simulink model "BAS_MPC_TV"  (R2018b)
settings: Solver=VariableStepAuto  StartTime=0.0  StopTime=10.0  RelTol=1e-3
values from neighbouring files (symbols this model uses):
  a = 1    [adaptive_mpc_tv.mat]
  b = 0.5    [adaptive_mpc_tv.mat]
  Izz = 100    [adaptive_mpc_tv.mat]
  M = 300    [adaptive_mpc_tv.mat]
  Rt = 0.226    [adaptive_mpc_tv.mat]
  track = 1.2    [adaptive_mpc_tv.mat]
  Ts = 0.02    [adaptive_mpc_tv.mat]
(part 2 of 2)

== system BAS_MPC_TV/For Iterator Subsystem1/function1/10layer_model/state_k_to_k+10 ==
  Fx : Inport
  Fy : Inport  Port=2
  statek : Inport  Port=3
  Add{,1,3..5,7} (6 alike) : Sum
  Add2 : Sum  Inputs=-+
  Add6 : Sum  Inputs=+--+-+
  Constant : Constant  Value=a
  Constant1 : Constant  Value=b
  Constant2 : Constant  Value=track
  Demux : Demux
  Demux1 : Demux
  Demux2 : Demux  Outputs=3
  Gain : Gain  Gain=0.5
  Multiply{,1..7} (8 alike) : Product
  Mux : Mux  Inputs=3
  Plus : Sum  Inputs=4
  Plus1 : Sum  Inputs=4
  Ts/Izz : Gain  Gain=Ts/Izz
  Ts/M : Gain  Gain=Ts/M
  Ts/M1 : Gain  Gain=Ts/M
  statek+1 : Outport
  wires:
  Demux2/2 -> Add3/1, Multiply/1
  Demux2/3 -> Multiply1/2, Multiply/2, Add7/1
  Multiply/1 -> Add/1
  Add/1 -> Ts/M/1
  Ts/M/1 -> Add1/2  "delta_Vx"
  Demux2/1 -> Add1/1, Multiply1/1
  Add1/1 -> Mux/1  "Vxk+1"
  Fx/1 -> Demux/1
  Demux/1 -> Multiply4/1, Plus/1  "Fx_FL"
  Demux/2 -> Multiply5/1, Plus/2  "Fx_FR"
  Demux/3 -> Multiply6/2, Plus/3  "Fx_RL"
  Demux/4 -> Plus/4, Multiply7/2  "Fx_RR"
  Plus/1 -> Add/2  "sumFx"
  Demux1/3 -> Add5/1, Plus1/3  "Fy_RL"
  Demux1/2 -> Add4/1, Plus1/2  "Fy_FR"
  Demux1/1 -> Add4/2, Plus1/1  "Fy_FL"
  Demux1/4 -> Add5/2, Plus1/4  "Fy_RR"
  Fy/1 -> Demux1/1
  Plus1/1 -> Add2/2  "sumFy"
  Multiply1/1 -> Add2/1
  Add2/1 -> Ts/M1/1
  Ts/M1/1 -> Add3/2  "delta_Vy"
  Add3/1 -> Mux/2  "Vyk+1"
  Add4/1 -> Multiply2/1
  Constant/1 -> Multiply2/2
  Multiply2/1 -> Add6/1
  Multiply3/1 -> Add6/2
  Constant1/1 -> Multiply3/2
  Add5/1 -> Multiply3/1
  Constant2/1 -> Gain/1
  Gain/1 -> Multiply7/1, Multiply4/2, Multiply5/2, Multiply6/1
  Multiply4/1 -> Add6/3
  Multiply5/1 -> Add6/4
  Multiply6/1 -> Add6/5
  Multiply7/1 -> Add6/6
  Add6/1 -> Ts/Izz/1
  Ts/Izz/1 -> Add7/2  "delta_yawrate"
  Add7/1 -> Mux/3  "yawratek+1"
  statek/1 -> Demux2/1
  Mux/1 -> statek+1/1

== system BAS_MPC_TV/For Iterator Subsystem1/function1/10layer_model/state_k_to_k+2 ==
  Fx : Inport
  Fy : Inport  Port=2
  statek : Inport  Port=3
  Add{,1,3..5,7} (6 alike) : Sum
  Add2 : Sum  Inputs=-+
  Add6 : Sum  Inputs=+--+-+
  Constant : Constant  Value=a
  Constant1 : Constant  Value=b
  Constant2 : Constant  Value=track
  Demux : Demux
  Demux1 : Demux
  Demux2 : Demux  Outputs=3
  Gain : Gain  Gain=0.5
  Multiply{,1..7} (8 alike) : Product
  Mux : Mux  Inputs=3
  Plus : Sum  Inputs=4
  Plus1 : Sum  Inputs=4
  Ts/Izz : Gain  Gain=Ts/Izz
  Ts/M : Gain  Gain=Ts/M
  Ts/M1 : Gain  Gain=Ts/M
  statek+1 : Outport
  wires:
  Demux2/2 -> Add3/1, Multiply/1
  Demux2/3 -> Multiply1/2, Multiply/2, Add7/1
  Multiply/1 -> Add/1
  Add/1 -> Ts/M/1
  Ts/M/1 -> Add1/2  "delta_Vx"
  Demux2/1 -> Add1/1, Multiply1/1
  Add1/1 -> Mux/1  "Vxk+1"
  Fx/1 -> Demux/1
  Demux/1 -> Multiply4/1, Plus/1  "Fx_FL"
  Demux/2 -> Multiply5/1, Plus/2  "Fx_FR"
  Demux/3 -> Multiply6/2, Plus/3  "Fx_RL"
  Demux/4 -> Plus/4, Multiply7/2  "Fx_RR"
  Plus/1 -> Add/2  "sumFx"
  Demux1/3 -> Add5/1, Plus1/3  "Fy_RL"
  Demux1/2 -> Add4/1, Plus1/2  "Fy_FR"
  Demux1/1 -> Add4/2, Plus1/1  "Fy_FL"
  Demux1/4 -> Add5/2, Plus1/4  "Fy_RR"
  Fy/1 -> Demux1/1
  Plus1/1 -> Add2/2  "sumFy"
  Multiply1/1 -> Add2/1
  Add2/1 -> Ts/M1/1
  Ts/M1/1 -> Add3/2  "delta_Vy"
  Add3/1 -> Mux/2  "Vyk+1"
  Add4/1 -> Multiply2/1
  Constant/1 -> Multiply2/2
  Multiply2/1 -> Add6/1
  Multiply3/1 -> Add6/2
  Constant1/1 -> Multiply3/2
  Add5/1 -> Multiply3/1
  Constant2/1 -> Gain/1
  Gain/1 -> Multiply7/1, Multiply4/2, Multiply5/2, Multiply6/1
  Multiply4/1 -> Add6/3
  Multiply5/1 -> Add6/4
  Multiply6/1 -> Add6/5
  Multiply7/1 -> Add6/6
  Add6/1 -> Ts/Izz/1
  Ts/Izz/1 -> Add7/2  "delta_yawrate"
  Add7/1 -> Mux/3  "yawratek+1"
  statek/1 -> Demux2/1
  Mux/1 -> statek+1/1

== system BAS_MPC_TV/For Iterator Subsystem1/function1/10layer_model/state_k_to_k+3 ==
  Fx : Inport
  Fy : Inport  Port=2
  statek : Inport  Port=3
  Add{,1,3..5,7} (6 alike) : Sum
  Add2 : Sum  Inputs=-+
  Add6 : Sum  Inputs=+--+-+
  Constant : Constant  Value=a
  Constant1 : Constant  Value=b
  Constant2 : Constant  Value=track
  Demux : Demux
  Demux1 : Demux
  Demux2 : Demux  Outputs=3
  Gain : Gain  Gain=0.5
  Multiply{,1..7} (8 alike) : Product
  Mux : Mux  Inputs=3
  Plus : Sum  Inputs=4
  Plus1 : Sum  Inputs=4
  Ts/Izz : Gain  Gain=Ts/Izz
  Ts/M : Gain  Gain=Ts/M
  Ts/M1 : Gain  Gain=Ts/M
  statek+1 : Outport
  wires:
  Demux2/2 -> Add3/1, Multiply/1
  Demux2/3 -> Multiply1/2, Multiply/2, Add7/1
  Multiply/1 -> Add/1
  Add/1 -> Ts/M/1
  Ts/M/1 -> Add1/2  "delta_Vx"
  Demux2/1 -> Add1/1, Multiply1/1
  Add1/1 -> Mux/1  "Vxk+1"
  Fx/1 -> Demux/1
  Demux/1 -> Multiply4/1, Plus/1  "Fx_FL"
  Demux/2 -> Multiply5/1, Plus/2  "Fx_FR"
  Demux/3 -> Multiply6/2, Plus/3  "Fx_RL"
  Demux/4 -> Plus/4, Multiply7/2  "Fx_RR"
  Plus/1 -> Add/2  "sumFx"
  Demux1/3 -> Add5/1, Plus1/3  "Fy_RL"
  Demux1/2 -> Add4/1, Plus1/2  "Fy_FR"
  Demux1/1 -> Add4/2, Plus1/1  "Fy_FL"
  Demux1/4 -> Add5/2, Plus1/4  "Fy_RR"
  Fy/1 -> Demux1/1
  Plus1/1 -> Add2/2  "sumFy"
  Multiply1/1 -> Add2/1
  Add2/1 -> Ts/M1/1
  Ts/M1/1 -> Add3/2  "delta_Vy"
  Add3/1 -> Mux/2  "Vyk+1"
  Add4/1 -> Multiply2/1
  Constant/1 -> Multiply2/2
  Multiply2/1 -> Add6/1
  Multiply3/1 -> Add6/2
  Constant1/1 -> Multiply3/2
  Add5/1 -> Multiply3/1
  Constant2/1 -> Gain/1
  Gain/1 -> Multiply7/1, Multiply4/2, Multiply5/2, Multiply6/1
  Multiply4/1 -> Add6/3
  Multiply5/1 -> Add6/4
  Multiply6/1 -> Add6/5
  Multiply7/1 -> Add6/6
  Add6/1 -> Ts/Izz/1
  Ts/Izz/1 -> Add7/2  "delta_yawrate"
  Add7/1 -> Mux/3  "yawratek+1"
  statek/1 -> Demux2/1
  Mux/1 -> statek+1/1

== system BAS_MPC_TV/For Iterator Subsystem1/function1/10layer_model/state_k_to_k+4 ==
  Fx : Inport
  Fy : Inport  Port=2
  statek : Inport  Port=3
  Add{,1,3..5,7} (6 alike) : Sum
  Add2 : Sum  Inputs=-+
  Add6 : Sum  Inputs=+--+-+
  Constant : Constant  Value=a
  Constant1 : Constant  Value=b
  Constant2 : Constant  Value=track
  Demux : Demux
  Demux1 : Demux
  Demux2 : Demux  Outputs=3
  Gain : Gain  Gain=0.5
  Multiply{,1..7} (8 alike) : Product
  Mux : Mux  Inputs=3
  Plus : Sum  Inputs=4
  Plus1 : Sum  Inputs=4
  Ts/Izz : Gain  Gain=Ts/Izz
  Ts/M : Gain  Gain=Ts/M
  Ts/M1 : Gain  Gain=Ts/M
  statek+1 : Outport
  wires:
  Demux2/2 -> Add3/1, Multiply/1
  Demux2/3 -> Multiply1/2, Multiply/2, Add7/1
  Multiply/1 -> Add/1
  Add/1 -> Ts/M/1
  Ts/M/1 -> Add1/2  "delta_Vx"
  Demux2/1 -> Add1/1, Multiply1/1
  Add1/1 -> Mux/1  "Vxk+1"
  Fx/1 -> Demux/1
  Demux/1 -> Multiply4/1, Plus/1  "Fx_FL"
  Demux/2 -> Multiply5/1, Plus/2  "Fx_FR"
  Demux/3 -> Multiply6/2, Plus/3  "Fx_RL"
  Demux/4 -> Plus/4, Multiply7/2  "Fx_RR"
  Plus/1 -> Add/2  "sumFx"
  Demux1/3 -> Add5/1, Plus1/3  "Fy_RL"
  Demux1/2 -> Add4/1, Plus1/2  "Fy_FR"
  Demux1/1 -> Add4/2, Plus1/1  "Fy_FL"
  Demux1/4 -> Add5/2, Plus1/4  "Fy_RR"
  Fy/1 -> Demux1/1
  Plus1/1 -> Add2/2  "sumFy"
  Multiply1/1 -> Add2/1
  Add2/1 -> Ts/M1/1
  Ts/M1/1 -> Add3/2  "delta_Vy"
  Add3/1 -> Mux/2  "Vyk+1"
  Add4/1 -> Multiply2/1
  Constant/1 -> Multiply2/2
  Multiply2/1 -> Add6/1
  Multiply3/1 -> Add6/2
  Constant1/1 -> Multiply3/2
  Add5/1 -> Multiply3/1
  Constant2/1 -> Gain/1
  Gain/1 -> Multiply7/1, Multiply4/2, Multiply5/2, Multiply6/1
  Multiply4/1 -> Add6/3
  Multiply5/1 -> Add6/4
  Multiply6/1 -> Add6/5
  Multiply7/1 -> Add6/6
  Add6/1 -> Ts/Izz/1
  Ts/Izz/1 -> Add7/2  "delta_yawrate"
  Add7/1 -> Mux/3  "yawratek+1"
  statek/1 -> Demux2/1
  Mux/1 -> statek+1/1

== system BAS_MPC_TV/For Iterator Subsystem1/function1/10layer_model/state_k_to_k+5 ==
  Fx : Inport
  Fy : Inport  Port=2
  statek : Inport  Port=3
  Add{,1,3..5,7} (6 alike) : Sum
  Add2 : Sum  Inputs=-+
  Add6 : Sum  Inputs=+--+-+
  Constant : Constant  Value=a
  Constant1 : Constant  Value=b
  Constant2 : Constant  Value=track
  Demux : Demux
  Demux1 : Demux
  Demux2 : Demux  Outputs=3
  Gain : Gain  Gain=0.5
  Multiply{,1..7} (8 alike) : Product
  Mux : Mux  Inputs=3
  Plus : Sum  Inputs=4
  Plus1 : Sum  Inputs=4
  Ts/Izz : Gain  Gain=Ts/Izz
  Ts/M : Gain  Gain=Ts/M
  Ts/M1 : Gain  Gain=Ts/M
  statek+1 : Outport
  wires:
  Demux2/2 -> Add3/1, Multiply/1
  Demux2/3 -> Multiply1/2, Multiply/2, Add7/1
  Multiply/1 -> Add/1
  Add/1 -> Ts/M/1
  Ts/M/1 -> Add1/2  "delta_Vx"
  Demux2/1 -> Add1/1, Multiply1/1
  Add1/1 -> Mux/1  "Vxk+1"
  Fx/1 -> Demux/1
  Demux/1 -> Multiply4/1, Plus/1  "Fx_FL"
  Demux/2 -> Multiply5/1, Plus/2  "Fx_FR"
  Demux/3 -> Multiply6/2, Plus/3  "Fx_RL"
  Demux/4 -> Plus/4, Multiply7/2  "Fx_RR"
  Plus/1 -> Add/2  "sumFx"
  Demux1/3 -> Add5/1, Plus1/3  "Fy_RL"
  Demux1/2 -> Add4/1, Plus1/2  "Fy_FR"
  Demux1/1 -> Add4/2, Plus1/1  "Fy_FL"
  Demux1/4 -> Add5/2, Plus1/4  "Fy_RR"
  Fy/1 -> Demux1/1
  Plus1/1 -> Add2/2  "sumFy"
  Multiply1/1 -> Add2/1
  Add2/1 -> Ts/M1/1
  Ts/M1/1 -> Add3/2  "delta_Vy"
  Add3/1 -> Mux/2  "Vyk+1"
  Add4/1 -> Multiply2/1
  Constant/1 -> Multiply2/2
  Multiply2/1 -> Add6/1
  Multiply3/1 -> Add6/2
  Constant1/1 -> Multiply3/2
  Add5/1 -> Multiply3/1
  Constant2/1 -> Gain/1
  Gain/1 -> Multiply7/1, Multiply4/2, Multiply5/2, Multiply6/1
  Multiply4/1 -> Add6/3
  Multiply5/1 -> Add6/4
  Multiply6/1 -> Add6/5
  Multiply7/1 -> Add6/6
  Add6/1 -> Ts/Izz/1
  Ts/Izz/1 -> Add7/2  "delta_yawrate"
  Add7/1 -> Mux/3  "yawratek+1"
  statek/1 -> Demux2/1
  Mux/1 -> statek+1/1

== system BAS_MPC_TV/For Iterator Subsystem1/function1/10layer_model/state_k_to_k+6 ==
  Fx : Inport
  Fy : Inport  Port=2
  statek : Inport  Port=3
  Add{,1,3..5,7} (6 alike) : Sum
  Add2 : Sum  Inputs=-+
  Add6 : Sum  Inputs=+--+-+
  Constant : Constant  Value=a
  Constant1 : Constant  Value=b
  Constant2 : Constant  Value=track
  Demux : Demux
  Demux1 : Demux
  Demux2 : Demux  Outputs=3
  Gain : Gain  Gain=0.5
  Multiply{,1..7} (8 alike) : Product
  Mux : Mux  Inputs=3
  Plus : Sum  Inputs=4
  Plus1 : Sum  Inputs=4
  Ts/Izz : Gain  Gain=Ts/Izz
  Ts/M : Gain  Gain=Ts/M
  Ts/M1 : Gain  Gain=Ts/M
  statek+1 : Outport
  wires:
  Demux2/2 -> Add3/1, Multiply/1
  Demux2/3 -> Multiply1/2, Multiply/2, Add7/1
  Multiply/1 -> Add/1
  Add/1 -> Ts/M/1
  Ts/M/1 -> Add1/2  "delta_Vx"
  Demux2/1 -> Add1/1, Multiply1/1
  Add1/1 -> Mux/1  "Vxk+1"
  Fx/1 -> Demux/1
  Demux/1 -> Multiply4/1, Plus/1  "Fx_FL"
  Demux/2 -> Multiply5/1, Plus/2  "Fx_FR"
  Demux/3 -> Multiply6/2, Plus/3  "Fx_RL"
  Demux/4 -> Plus/4, Multiply7/2  "Fx_RR"
  Plus/1 -> Add/2  "sumFx"
  Demux1/3 -> Add5/1, Plus1/3  "Fy_RL"
  Demux1/2 -> Add4/1, Plus1/2  "Fy_FR"
  Demux1/1 -> Add4/2, Plus1/1  "Fy_FL"
  Demux1/4 -> Add5/2, Plus1/4  "Fy_RR"
  Fy/1 -> Demux1/1
  Plus1/1 -> Add2/2  "sumFy"
  Multiply1/1 -> Add2/1
  Add2/1 -> Ts/M1/1
  Ts/M1/1 -> Add3/2  "delta_Vy"
  Add3/1 -> Mux/2  "Vyk+1"
  Add4/1 -> Multiply2/1
  Constant/1 -> Multiply2/2
  Multiply2/1 -> Add6/1
  Multiply3/1 -> Add6/2
  Constant1/1 -> Multiply3/2
  Add5/1 -> Multiply3/1
  Constant2/1 -> Gain/1
  Gain/1 -> Multiply7/1, Multiply4/2, Multiply5/2, Multiply6/1
  Multiply4/1 -> Add6/3
  Multiply5/1 -> Add6/4
  Multiply6/1 -> Add6/5
  Multiply7/1 -> Add6/6
  Add6/1 -> Ts/Izz/1
  Ts/Izz/1 -> Add7/2  "delta_yawrate"
  Add7/1 -> Mux/3  "yawratek+1"
  statek/1 -> Demux2/1
  Mux/1 -> statek+1/1

== system BAS_MPC_TV/For Iterator Subsystem1/function1/10layer_model/state_k_to_k+7 ==
  Fx : Inport
  Fy : Inport  Port=2
  statek : Inport  Port=3
  Add{,1,3..5,7} (6 alike) : Sum
  Add2 : Sum  Inputs=-+
  Add6 : Sum  Inputs=+--+-+
  Constant : Constant  Value=a
  Constant1 : Constant  Value=b
  Constant2 : Constant  Value=track
  Demux : Demux
  Demux1 : Demux
  Demux2 : Demux  Outputs=3
  Gain : Gain  Gain=0.5
  Multiply{,1..7} (8 alike) : Product
  Mux : Mux  Inputs=3
  Plus : Sum  Inputs=4
  Plus1 : Sum  Inputs=4
  Ts/Izz : Gain  Gain=Ts/Izz
  Ts/M : Gain  Gain=Ts/M
  Ts/M1 : Gain  Gain=Ts/M
  statek+1 : Outport
  wires:
  Demux2/2 -> Add3/1, Multiply/1
  Demux2/3 -> Multiply1/2, Multiply/2, Add7/1
  Multiply/1 -> Add/1
  Add/1 -> Ts/M/1
  Ts/M/1 -> Add1/2  "delta_Vx"
  Demux2/1 -> Add1/1, Multiply1/1
  Add1/1 -> Mux/1  "Vxk+1"
  Fx/1 -> Demux/1
  Demux/1 -> Multiply4/1, Plus/1  "Fx_FL"
  Demux/2 -> Multiply5/1, Plus/2  "Fx_FR"
  Demux/3 -> Multiply6/2, Plus/3  "Fx_RL"
  Demux/4 -> Plus/4, Multiply7/2  "Fx_RR"
  Plus/1 -> Add/2  "sumFx"
  Demux1/3 -> Add5/1, Plus1/3  "Fy_RL"
  Demux1/2 -> Add4/1, Plus1/2  "Fy_FR"
  Demux1/1 -> Add4/2, Plus1/1  "Fy_FL"
  Demux1/4 -> Add5/2, Plus1/4  "Fy_RR"
  Fy/1 -> Demux1/1
  Plus1/1 -> Add2/2  "sumFy"
  Multiply1/1 -> Add2/1
  Add2/1 -> Ts/M1/1
  Ts/M1/1 -> Add3/2  "delta_Vy"
  Add3/1 -> Mux/2  "Vyk+1"
  Add4/1 -> Multiply2/1
  Constant/1 -> Multiply2/2
  Multiply2/1 -> Add6/1
  Multiply3/1 -> Add6/2
  Constant1/1 -> Multiply3/2
  Add5/1 -> Multiply3/1
  Constant2/1 -> Gain/1
  Gain/1 -> Multiply7/1, Multiply4/2, Multiply5/2, Multiply6/1
  Multiply4/1 -> Add6/3
  Multiply5/1 -> Add6/4
  Multiply6/1 -> Add6/5
  Multiply7/1 -> Add6/6
  Add6/1 -> Ts/Izz/1
  Ts/Izz/1 -> Add7/2  "delta_yawrate"
  Add7/1 -> Mux/3  "yawratek+1"
  statek/1 -> Demux2/1
  Mux/1 -> statek+1/1

== system BAS_MPC_TV/For Iterator Subsystem1/function1/10layer_model/state_k_to_k+8 ==
  Fx : Inport
  Fy : Inport  Port=2
  statek : Inport  Port=3
  Add{,1,3..5,7} (6 alike) : Sum
  Add2 : Sum  Inputs=-+
  Add6 : Sum  Inputs=+--+-+
  Constant : Constant  Value=a
  Constant1 : Constant  Value=b
  Constant2 : Constant  Value=track
  Demux : Demux
  Demux1 : Demux
  Demux2 : Demux  Outputs=3
  Gain : Gain  Gain=0.5
  Multiply{,1..7} (8 alike) : Product
  Mux : Mux  Inputs=3
  Plus : Sum  Inputs=4
  Plus1 : Sum  Inputs=4
  Ts/Izz : Gain  Gain=Ts/Izz
  Ts/M : Gain  Gain=Ts/M
  Ts/M1 : Gain  Gain=Ts/M
  statek+1 : Outport
  wires:
  Demux2/2 -> Add3/1, Multiply/1
  Demux2/3 -> Multiply1/2, Multiply/2, Add7/1
  Multiply/1 -> Add/1
  Add/1 -> Ts/M/1
  Ts/M/1 -> Add1/2  "delta_Vx"
  Demux2/1 -> Add1/1, Multiply1/1
  Add1/1 -> Mux/1  "Vxk+1"
  Fx/1 -> Demux/1
  Demux/1 -> Multiply4/1, Plus/1  "Fx_FL"
  Demux/2 -> Multiply5/1, Plus/2  "Fx_FR"
  Demux/3 -> Multiply6/2, Plus/3  "Fx_RL"
  Demux/4 -> Plus/4, Multiply7/2  "Fx_RR"
  Plus/1 -> Add/2  "sumFx"
  Demux1/3 -> Add5/1, Plus1/3  "Fy_RL"
  Demux1/2 -> Add4/1, Plus1/2  "Fy_FR"
  Demux1/1 -> Add4/2, Plus1/1  "Fy_FL"
  Demux1/4 -> Add5/2, Plus1/4  "Fy_RR"
  Fy/1 -> Demux1/1
  Plus1/1 -> Add2/2  "sumFy"
  Multiply1/1 -> Add2/1
  Add2/1 -> Ts/M1/1
  Ts/M1/1 -> Add3/2  "delta_Vy"
  Add3/1 -> Mux/2  "Vyk+1"
  Add4/1 -> Multiply2/1
  Constant/1 -> Multiply2/2
  Multiply2/1 -> Add6/1
  Multiply3/1 -> Add6/2
  Constant1/1 -> Multiply3/2
  Add5/1 -> Multiply3/1
  Constant2/1 -> Gain/1
  Gain/1 -> Multiply7/1, Multiply4/2, Multiply5/2, Multiply6/1
  Multiply4/1 -> Add6/3
  Multiply5/1 -> Add6/4
  Multiply6/1 -> Add6/5
  Multiply7/1 -> Add6/6
  Add6/1 -> Ts/Izz/1
  Ts/Izz/1 -> Add7/2  "delta_yawrate"
  Add7/1 -> Mux/3  "yawratek+1"
  statek/1 -> Demux2/1
  Mux/1 -> statek+1/1

== system BAS_MPC_TV/For Iterator Subsystem1/function1/10layer_model/state_k_to_k+9 ==
  Fx : Inport
  Fy : Inport  Port=2
  statek : Inport  Port=3
  Add{,1,3..5,7} (6 alike) : Sum
  Add2 : Sum  Inputs=-+
  Add6 : Sum  Inputs=+--+-+
  Constant : Constant  Value=a
  Constant1 : Constant  Value=b
  Constant2 : Constant  Value=track
  Demux : Demux
  Demux1 : Demux
  Demux2 : Demux  Outputs=3
  Gain : Gain  Gain=0.5
  Multiply{,1..7} (8 alike) : Product
  Mux : Mux  Inputs=3
  Plus : Sum  Inputs=4
  Plus1 : Sum  Inputs=4
  Ts/Izz : Gain  Gain=Ts/Izz
  Ts/M : Gain  Gain=Ts/M
  Ts/M1 : Gain  Gain=Ts/M
  statek+1 : Outport
  wires:
  Demux2/2 -> Add3/1, Multiply/1
  Demux2/3 -> Multiply1/2, Multiply/2, Add7/1
  Multiply/1 -> Add/1
  Add/1 -> Ts/M/1
  Ts/M/1 -> Add1/2  "delta_Vx"
  Demux2/1 -> Add1/1, Multiply1/1
  Add1/1 -> Mux/1  "Vxk+1"
  Fx/1 -> Demux/1
  Demux/1 -> Multiply4/1, Plus/1  "Fx_FL"
  Demux/2 -> Multiply5/1, Plus/2  "Fx_FR"
  Demux/3 -> Multiply6/2, Plus/3  "Fx_RL"
  Demux/4 -> Plus/4, Multiply7/2  "Fx_RR"
  Plus/1 -> Add/2  "sumFx"
  Demux1/3 -> Add5/1, Plus1/3  "Fy_RL"
  Demux1/2 -> Add4/1, Plus1/2  "Fy_FR"
  Demux1/1 -> Add4/2, Plus1/1  "Fy_FL"
  Demux1/4 -> Add5/2, Plus1/4  "Fy_RR"
  Fy/1 -> Demux1/1
  Plus1/1 -> Add2/2  "sumFy"
  Multiply1/1 -> Add2/1
  Add2/1 -> Ts/M1/1
  Ts/M1/1 -> Add3/2  "delta_Vy"
  Add3/1 -> Mux/2  "Vyk+1"
  Add4/1 -> Multiply2/1
  Constant/1 -> Multiply2/2
  Multiply2/1 -> Add6/1
  Multiply3/1 -> Add6/2
  Constant1/1 -> Multiply3/2
  Add5/1 -> Multiply3/1
  Constant2/1 -> Gain/1
  Gain/1 -> Multiply7/1, Multiply4/2, Multiply5/2, Multiply6/1
  Multiply4/1 -> Add6/3
  Multiply5/1 -> Add6/4
  Multiply6/1 -> Add6/5
  Multiply7/1 -> Add6/6
  Add6/1 -> Ts/Izz/1
  Ts/Izz/1 -> Add7/2  "delta_yawrate"
  Add7/1 -> Mux/3  "yawratek+1"
  statek/1 -> Demux2/1
  Mux/1 -> statek+1/1

== system BAS_MPC_TV/For Iterator Subsystem1/function2/10layer_model/state_k_to_k+1 ==
  Fx : Inport
  Fy : Inport  Port=2
  statek : Inport  Port=3
  Add{,1,3..5,7} (6 alike) : Sum
  Add2 : Sum  Inputs=-+
  Add6 : Sum  Inputs=+--+-+
  Constant : Constant  Value=a
  Constant1 : Constant  Value=b
  Constant2 : Constant  Value=track
  Demux : Demux
  Demux1 : Demux
  Demux2 : Demux  Outputs=3
  Gain : Gain  Gain=0.5
  Multiply{,1..7} (8 alike) : Product
  Mux : Mux  Inputs=3
  Plus : Sum  Inputs=4
  Plus1 : Sum  Inputs=4
  Ts/Izz : Gain  Gain=Ts/Izz
  Ts/M : Gain  Gain=Ts/M
  Ts/M1 : Gain  Gain=Ts/M
  statek+1 : Outport
  wires:
  Demux2/2 -> Add3/1, Multiply/1
  Demux2/3 -> Multiply1/2, Multiply/2, Add7/1
  Multiply/1 -> Add/1
  Add/1 -> Ts/M/1
  Ts/M/1 -> Add1/2  "delta_Vx"
  Demux2/1 -> Add1/1, Multiply1/1
  Add1/1 -> Mux/1  "Vxk+1"
  Fx/1 -> Demux/1
  Demux/1 -> Multiply4/1, Plus/1  "Fx_FL"
  Demux/2 -> Multiply5/1, Plus/2  "Fx_FR"
  Demux/3 -> Multiply6/2, Plus/3  "Fx_RL"
  Demux/4 -> Plus/4, Multiply7/2  "Fx_RR"
  Plus/1 -> Add/2  "sumFx"
  Demux1/3 -> Add5/1, Plus1/3  "Fy_RL"
  Demux1/2 -> Add4/1, Plus1/2  "Fy_FR"
  Demux1/1 -> Add4/2, Plus1/1  "Fy_FL"
  Demux1/4 -> Add5/2, Plus1/4  "Fy_RR"
  Fy/1 -> Demux1/1
  Plus1/1 -> Add2/2  "sumFy"
  Multiply1/1 -> Add2/1
  Add2/1 -> Ts/M1/1
  Ts/M1/1 -> Add3/2  "delta_Vy"
  Add3/1 -> Mux/2  "Vyk+1"
  Add4/1 -> Multiply2/1
  Constant/1 -> Multiply2/2
  Multiply2/1 -> Add6/1
  Multiply3/1 -> Add6/2
  Constant1/1 -> Multiply3/2
  Add5/1 -> Multiply3/1
  Constant2/1 -> Gain/1
  Gain/1 -> Multiply7/1, Multiply4/2, Multiply5/2, Multiply6/1
  Multiply4/1 -> Add6/3
  Multiply5/1 -> Add6/4
  Multiply6/1 -> Add6/5
  Multiply7/1 -> Add6/6
  Add6/1 -> Ts/Izz/1
  Ts/Izz/1 -> Add7/2  "delta_yawrate"
  Add7/1 -> Mux/3  "yawratek+1"
  statek/1 -> Demux2/1
  Mux/1 -> statek+1/1

== system BAS_MPC_TV/For Iterator Subsystem1/function2/10layer_model/state_k_to_k+10 ==
  Fx : Inport
  Fy : Inport  Port=2
  statek : Inport  Port=3
  Add{,1,3..5,7} (6 alike) : Sum
  Add2 : Sum  Inputs=-+
  Add6 : Sum  Inputs=+--+-+
  Constant : Constant  Value=a
  Constant1 : Constant  Value=b
  Constant2 : Constant  Value=track
  Demux : Demux
  Demux1 : Demux
  Demux2 : Demux  Outputs=3
  Gain : Gain  Gain=0.5
  Multiply{,1..7} (8 alike) : Product
  Mux : Mux  Inputs=3
  Plus : Sum  Inputs=4
  Plus1 : Sum  Inputs=4
  Ts/Izz : Gain  Gain=Ts/Izz
  Ts/M : Gain  Gain=Ts/M
  Ts/M1 : Gain  Gain=Ts/M
  statek+1 : Outport
  wires:
  Demux2/2 -> Add3/1, Multiply/1
  Demux2/3 -> Multiply1/2, Multiply/2, Add7/1
  Multiply/1 -> Add/1
  Add/1 -> Ts/M/1
  Ts/M/1 -> Add1/2  "delta_Vx"
  Demux2/1 -> Add1/1, Multiply1/1
  Add1/1 -> Mux/1  "Vxk+1"
  Fx/1 -> Demux/1
  Demux/1 -> Multiply4/1, Plus/1  "Fx_FL"
  Demux/2 -> Multiply5/1, Plus/2  "Fx_FR"
  Demux/3 -> Multiply6/2, Plus/3  "Fx_RL"
  Demux/4 -> Plus/4, Multiply7/2  "Fx_RR"
  Plus/1 -> Add/2  "sumFx"
  Demux1/3 -> Add5/1, Plus1/3  "Fy_RL"
  Demux1/2 -> Add4/1, Plus1/2  "Fy_FR"
  Demux1/1 -> Add4/2, Plus1/1  "Fy_FL"
  Demux1/4 -> Add5/2, Plus1/4  "Fy_RR"
  Fy/1 -> Demux1/1
  Plus1/1 -> Add2/2  "sumFy"
  Multiply1/1 -> Add2/1
  Add2/1 -> Ts/M1/1
  Ts/M1/1 -> Add3/2  "delta_Vy"
  Add3/1 -> Mux/2  "Vyk+1"
  Add4/1 -> Multiply2/1
  Constant/1 -> Multiply2/2
  Multiply2/1 -> Add6/1
  Multiply3/1 -> Add6/2
  Constant1/1 -> Multiply3/2
  Add5/1 -> Multiply3/1
  Constant2/1 -> Gain/1
  Gain/1 -> Multiply7/1, Multiply4/2, Multiply5/2, Multiply6/1
  Multiply4/1 -> Add6/3
  Multiply5/1 -> Add6/4
  Multiply6/1 -> Add6/5
  Multiply7/1 -> Add6/6
  Add6/1 -> Ts/Izz/1
  Ts/Izz/1 -> Add7/2  "delta_yawrate"
  Add7/1 -> Mux/3  "yawratek+1"
  statek/1 -> Demux2/1
  Mux/1 -> statek+1/1

== system BAS_MPC_TV/For Iterator Subsystem1/function2/10layer_model/state_k_to_k+2 ==
  Fx : Inport
  Fy : Inport  Port=2
  statek : Inport  Port=3
  Add{,1,3..5,7} (6 alike) : Sum
  Add2 : Sum  Inputs=-+
  Add6 : Sum  Inputs=+--+-+
  Constant : Constant  Value=a
  Constant1 : Constant  Value=b
  Constant2 : Constant  Value=track
  Demux : Demux
  Demux1 : Demux
  Demux2 : Demux  Outputs=3
  Gain : Gain  Gain=0.5
  Multiply{,1..7} (8 alike) : Product
  Mux : Mux  Inputs=3
  Plus : Sum  Inputs=4
  Plus1 : Sum  Inputs=4
  Ts/Izz : Gain  Gain=Ts/Izz
  Ts/M : Gain  Gain=Ts/M
  Ts/M1 : Gain  Gain=Ts/M
  statek+1 : Outport
  wires:
  Demux2/2 -> Add3/1, Multiply/1
  Demux2/3 -> Multiply1/2, Multiply/2, Add7/1
  Multiply/1 -> Add/1
  Add/1 -> Ts/M/1
  Ts/M/1 -> Add1/2  "delta_Vx"
  Demux2/1 -> Add1/1, Multiply1/1
  Add1/1 -> Mux/1  "Vxk+1"
  Fx/1 -> Demux/1
  Demux/1 -> Multiply4/1, Plus/1  "Fx_FL"
  Demux/2 -> Multiply5/1, Plus/2  "Fx_FR"
  Demux/3 -> Multiply6/2, Plus/3  "Fx_RL"
  Demux/4 -> Plus/4, Multiply7/2  "Fx_RR"
  Plus/1 -> Add/2  "sumFx"
  Demux1/3 -> Add5/1, Plus1/3  "Fy_RL"
  Demux1/2 -> Add4/1, Plus1/2  "Fy_FR"
  Demux1/1 -> Add4/2, Plus1/1  "Fy_FL"
  Demux1/4 -> Add5/2, Plus1/4  "Fy_RR"
  Fy/1 -> Demux1/1
  Plus1/1 -> Add2/2  "sumFy"
  Multiply1/1 -> Add2/1
  Add2/1 -> Ts/M1/1
  Ts/M1/1 -> Add3/2  "delta_Vy"
  Add3/1 -> Mux/2  "Vyk+1"
  Add4/1 -> Multiply2/1
  Constant/1 -> Multiply2/2
  Multiply2/1 -> Add6/1
  Multiply3/1 -> Add6/2
  Constant1/1 -> Multiply3/2
  Add5/1 -> Multiply3/1
  Constant2/1 -> Gain/1
  Gain/1 -> Multiply7/1, Multiply4/2, Multiply5/2, Multiply6/1
  Multiply4/1 -> Add6/3
  Multiply5/1 -> Add6/4
  Multiply6/1 -> Add6/5
  Multiply7/1 -> Add6/6
  Add6/1 -> Ts/Izz/1
  Ts/Izz/1 -> Add7/2  "delta_yawrate"
  Add7/1 -> Mux/3  "yawratek+1"
  statek/1 -> Demux2/1
  Mux/1 -> statek+1/1

== system BAS_MPC_TV/For Iterator Subsystem1/function2/10layer_model/state_k_to_k+3 ==
  Fx : Inport
  Fy : Inport  Port=2
  statek : Inport  Port=3
  Add{,1,3..5,7} (6 alike) : Sum
  Add2 : Sum  Inputs=-+
  Add6 : Sum  Inputs=+--+-+
  Constant : Constant  Value=a
  Constant1 : Constant  Value=b
  Constant2 : Constant  Value=track
  Demux : Demux
  Demux1 : Demux
  Demux2 : Demux  Outputs=3
  Gain : Gain  Gain=0.5
  Multiply{,1..7} (8 alike) : Product
  Mux : Mux  Inputs=3
  Plus : Sum  Inputs=4
  Plus1 : Sum  Inputs=4
  Ts/Izz : Gain  Gain=Ts/Izz
  Ts/M : Gain  Gain=Ts/M
  Ts/M1 : Gain  Gain=Ts/M
  statek+1 : Outport
  wires:
  Demux2/2 -> Add3/1, Multiply/1
  Demux2/3 -> Multiply1/2, Multiply/2, Add7/1
  Multiply/1 -> Add/1
  Add/1 -> Ts/M/1
  Ts/M/1 -> Add1/2  "delta_Vx"
  Demux2/1 -> Add1/1, Multiply1/1
  Add1/1 -> Mux/1  "Vxk+1"
  Fx/1 -> Demux/1
  Demux/1 -> Multiply4/1, Plus/1  "Fx_FL"
  Demux/2 -> Multiply5/1, Plus/2  "Fx_FR"
  Demux/3 -> Multiply6/2, Plus/3  "Fx_RL"
  Demux/4 -> Plus/4, Multiply7/2  "Fx_RR"
  Plus/1 -> Add/2  "sumFx"
  Demux1/3 -> Add5/1, Plus1/3  "Fy_RL"
  Demux1/2 -> Add4/1, Plus1/2  "Fy_FR"
  Demux1/1 -> Add4/2, Plus1/1  "Fy_FL"
  Demux1/4 -> Add5/2, Plus1/4  "Fy_RR"
  Fy/1 -> Demux1/1
  Plus1/1 -> Add2/2  "sumFy"
  Multiply1/1 -> Add2/1
  Add2/1 -> Ts/M1/1
  Ts/M1/1 -> Add3/2  "delta_Vy"
  Add3/1 -> Mux/2  "Vyk+1"
  Add4/1 -> Multiply2/1
  Constant/1 -> Multiply2/2
  Multiply2/1 -> Add6/1
  Multiply3/1 -> Add6/2
  Constant1/1 -> Multiply3/2
  Add5/1 -> Multiply3/1
  Constant2/1 -> Gain/1
  Gain/1 -> Multiply7/1, Multiply4/2, Multiply5/2, Multiply6/1
  Multiply4/1 -> Add6/3
  Multiply5/1 -> Add6/4
  Multiply6/1 -> Add6/5
  Multiply7/1 -> Add6/6
  Add6/1 -> Ts/Izz/1
  Ts/Izz/1 -> Add7/2  "delta_yawrate"
  Add7/1 -> Mux/3  "yawratek+1"
  statek/1 -> Demux2/1
  Mux/1 -> statek+1/1

== system BAS_MPC_TV/For Iterator Subsystem1/function2/10layer_model/state_k_to_k+4 ==
  Fx : Inport
  Fy : Inport  Port=2
  statek : Inport  Port=3
  Add{,1,3..5,7} (6 alike) : Sum
  Add2 : Sum  Inputs=-+
  Add6 : Sum  Inputs=+--+-+
  Constant : Constant  Value=a
  Constant1 : Constant  Value=b
  Constant2 : Constant  Value=track
  Demux : Demux
  Demux1 : Demux
  Demux2 : Demux  Outputs=3
  Gain : Gain  Gain=0.5
  Multiply{,1..7} (8 alike) : Product
  Mux : Mux  Inputs=3
  Plus : Sum  Inputs=4
  Plus1 : Sum  Inputs=4
  Ts/Izz : Gain  Gain=Ts/Izz
  Ts/M : Gain  Gain=Ts/M
  Ts/M1 : Gain  Gain=Ts/M
  statek+1 : Outport
  wires:
  Demux2/2 -> Add3/1, Multiply/1
  Demux2/3 -> Multiply1/2, Multiply/2, Add7/1
  Multiply/1 -> Add/1
  Add/1 -> Ts/M/1
  Ts/M/1 -> Add1/2  "delta_Vx"
  Demux2/1 -> Add1/1, Multiply1/1
  Add1/1 -> Mux/1  "Vxk+1"
  Fx/1 -> Demux/1
  Demux/1 -> Multiply4/1, Plus/1  "Fx_FL"
  Demux/2 -> Multiply5/1, Plus/2  "Fx_FR"
  Demux/3 -> Multiply6/2, Plus/3  "Fx_RL"
  Demux/4 -> Plus/4, Multiply7/2  "Fx_RR"
  Plus/1 -> Add/2  "sumFx"
  Demux1/3 -> Add5/1, Plus1/3  "Fy_RL"
  Demux1/2 -> Add4/1, Plus1/2  "Fy_FR"
  Demux1/1 -> Add4/2, Plus1/1  "Fy_FL"
  Demux1/4 -> Add5/2, Plus1/4  "Fy_RR"
  Fy/1 -> Demux1/1
  Plus1/1 -> Add2/2  "sumFy"
  Multiply1/1 -> Add2/1
  Add2/1 -> Ts/M1/1
  Ts/M1/1 -> Add3/2  "delta_Vy"
  Add3/1 -> Mux/2  "Vyk+1"
  Add4/1 -> Multiply2/1
  Constant/1 -> Multiply2/2
  Multiply2/1 -> Add6/1
  Multiply3/1 -> Add6/2
  Constant1/1 -> Multiply3/2
  Add5/1 -> Multiply3/1
  Constant2/1 -> Gain/1
  Gain/1 -> Multiply7/1, Multiply4/2, Multiply5/2, Multiply6/1
  Multiply4/1 -> Add6/3
  Multiply5/1 -> Add6/4
  Multiply6/1 -> Add6/5
  Multiply7/1 -> Add6/6
  Add6/1 -> Ts/Izz/1
  Ts/Izz/1 -> Add7/2  "delta_yawrate"
  Add7/1 -> Mux/3  "yawratek+1"
  statek/1 -> Demux2/1
  Mux/1 -> statek+1/1

== system BAS_MPC_TV/For Iterator Subsystem1/function2/10layer_model/state_k_to_k+5 ==
  Fx : Inport
  Fy : Inport  Port=2
  statek : Inport  Port=3
  Add{,1,3..5,7} (6 alike) : Sum
  Add2 : Sum  Inputs=-+
  Add6 : Sum  Inputs=+--+-+
  Constant : Constant  Value=a
  Constant1 : Constant  Value=b
  Constant2 : Constant  Value=track
  Demux : Demux
  Demux1 : Demux
  Demux2 : Demux  Outputs=3
  Gain : Gain  Gain=0.5
  Multiply{,1..7} (8 alike) : Product
  Mux : Mux  Inputs=3
  Plus : Sum  Inputs=4
  Plus1 : Sum  Inputs=4
  Ts/Izz : Gain  Gain=Ts/Izz
  Ts/M : Gain  Gain=Ts/M
  Ts/M1 : Gain  Gain=Ts/M
  statek+1 : Outport
  wires:
  Demux2/2 -> Add3/1, Multiply/1
  Demux2/3 -> Multiply1/2, Multiply/2, Add7/1
  Multiply/1 -> Add/1
  Add/1 -> Ts/M/1
  Ts/M/1 -> Add1/2  "delta_Vx"
  Demux2/1 -> Add1/1, Multiply1/1
  Add1/1 -> Mux/1  "Vxk+1"
  Fx/1 -> Demux/1
  Demux/1 -> Multiply4/1, Plus/1  "Fx_FL"
  Demux/2 -> Multiply5/1, Plus/2  "Fx_FR"
  Demux/3 -> Multiply6/2, Plus/3  "Fx_RL"
  Demux/4 -> Plus/4, Multiply7/2  "Fx_RR"
  Plus/1 -> Add/2  "sumFx"
  Demux1/3 -> Add5/1, Plus1/3  "Fy_RL"
  Demux1/2 -> Add4/1, Plus1/2  "Fy_FR"
  Demux1/1 -> Add4/2, Plus1/1  "Fy_FL"
  Demux1/4 -> Add5/2, Plus1/4  "Fy_RR"
  Fy/1 -> Demux1/1
  Plus1/1 -> Add2/2  "sumFy"
  Multiply1/1 -> Add2/1
  Add2/1 -> Ts/M1/1
  Ts/M1/1 -> Add3/2  "delta_Vy"
  Add3/1 -> Mux/2  "Vyk+1"
  Add4/1 -> Multiply2/1
  Constant/1 -> Multiply2/2
  Multiply2/1 -> Add6/1
  Multiply3/1 -> Add6/2
  Constant1/1 -> Multiply3/2
  Add5/1 -> Multiply3/1
  Constant2/1 -> Gain/1
  Gain/1 -> Multiply7/1, Multiply4/2, Multiply5/2, Multiply6/1
  Multiply4/1 -> Add6/3
  Multiply5/1 -> Add6/4
  Multiply6/1 -> Add6/5
  Multiply7/1 -> Add6/6
  Add6/1 -> Ts/Izz/1
  Ts/Izz/1 -> Add7/2  "delta_yawrate"
  Add7/1 -> Mux/3  "yawratek+1"
  statek/1 -> Demux2/1
  Mux/1 -> statek+1/1

== system BAS_MPC_TV/For Iterator Subsystem1/function2/10layer_model/state_k_to_k+6 ==
  Fx : Inport
  Fy : Inport  Port=2
  statek : Inport  Port=3
  Add{,1,3..5,7} (6 alike) : Sum
  Add2 : Sum  Inputs=-+
  Add6 : Sum  Inputs=+--+-+
  Constant : Constant  Value=a
  Constant1 : Constant  Value=b
  Constant2 : Constant  Value=track
  Demux : Demux
  Demux1 : Demux
  Demux2 : Demux  Outputs=3
  Gain : Gain  Gain=0.5
  Multiply{,1..7} (8 alike) : Product
  Mux : Mux  Inputs=3
  Plus : Sum  Inputs=4
  Plus1 : Sum  Inputs=4
  Ts/Izz : Gain  Gain=Ts/Izz
  Ts/M : Gain  Gain=Ts/M
  Ts/M1 : Gain  Gain=Ts/M
  statek+1 : Outport
  wires:
  Demux2/2 -> Add3/1, Multiply/1
  Demux2/3 -> Multiply1/2, Multiply/2, Add7/1
  Multiply/1 -> Add/1
  Add/1 -> Ts/M/1
  Ts/M/1 -> Add1/2  "delta_Vx"
  Demux2/1 -> Add1/1, Multiply1/1
  Add1/1 -> Mux/1  "Vxk+1"
  Fx/1 -> Demux/1
  Demux/1 -> Multiply4/1, Plus/1  "Fx_FL"
  Demux/2 -> Multiply5/1, Plus/2  "Fx_FR"
  Demux/3 -> Multiply6/2, Plus/3  "Fx_RL"
  Demux/4 -> Plus/4, Multiply7/2  "Fx_RR"
  Plus/1 -> Add/2  "sumFx"
  Demux1/3 -> Add5/1, Plus1/3  "Fy_RL"
  Demux1/2 -> Add4/1, Plus1/2  "Fy_FR"
  Demux1/1 -> Add4/2, Plus1/1  "Fy_FL"
  Demux1/4 -> Add5/2, Plus1/4  "Fy_RR"
  Fy/1 -> Demux1/1
  Plus1/1 -> Add2/2  "sumFy"
  Multiply1/1 -> Add2/1
  Add2/1 -> Ts/M1/1
  Ts/M1/1 -> Add3/2  "delta_Vy"
  Add3/1 -> Mux/2  "Vyk+1"
  Add4/1 -> Multiply2/1
  Constant/1 -> Multiply2/2
  Multiply2/1 -> Add6/1
  Multiply3/1 -> Add6/2
  Constant1/1 -> Multiply3/2
  Add5/1 -> Multiply3/1
  Constant2/1 -> Gain/1
  Gain/1 -> Multiply7/1, Multiply4/2, Multiply5/2, Multiply6/1
  Multiply4/1 -> Add6/3
  Multiply5/1 -> Add6/4
  Multiply6/1 -> Add6/5
  Multiply7/1 -> Add6/6
  Add6/1 -> Ts/Izz/1
  Ts/Izz/1 -> Add7/2  "delta_yawrate"
  Add7/1 -> Mux/3  "yawratek+1"
  statek/1 -> Demux2/1
  Mux/1 -> statek+1/1

== system BAS_MPC_TV/For Iterator Subsystem1/function2/10layer_model/state_k_to_k+7 ==
  Fx : Inport
  Fy : Inport  Port=2
  statek : Inport  Port=3
  Add{,1,3..5,7} (6 alike) : Sum
  Add2 : Sum  Inputs=-+
  Add6 : Sum  Inputs=+--+-+
  Constant : Constant  Value=a
  Constant1 : Constant  Value=b
  Constant2 : Constant  Value=track
  Demux : Demux
  Demux1 : Demux
  Demux2 : Demux  Outputs=3
  Gain : Gain  Gain=0.5
  Multiply{,1..7} (8 alike) : Product
  Mux : Mux  Inputs=3
  Plus : Sum  Inputs=4
  Plus1 : Sum  Inputs=4
  Ts/Izz : Gain  Gain=Ts/Izz
  Ts/M : Gain  Gain=Ts/M
  Ts/M1 : Gain  Gain=Ts/M
  statek+1 : Outport
  wires:
  Demux2/2 -> Add3/1, Multiply/1
  Demux2/3 -> Multiply1/2, Multiply/2, Add7/1
  Multiply/1 -> Add/1
  Add/1 -> Ts/M/1
  Ts/M/1 -> Add1/2  "delta_Vx"
  Demux2/1 -> Add1/1, Multiply1/1
  Add1/1 -> Mux/1  "Vxk+1"
  Fx/1 -> Demux/1
  Demux/1 -> Multiply4/1, Plus/1  "Fx_FL"
  Demux/2 -> Multiply5/1, Plus/2  "Fx_FR"
  Demux/3 -> Multiply6/2, Plus/3  "Fx_RL"
  Demux/4 -> Plus/4, Multiply7/2  "Fx_RR"
  Plus/1 -> Add/2  "sumFx"
  Demux1/3 -> Add5/1, Plus1/3  "Fy_RL"
  Demux1/2 -> Add4/1, Plus1/2  "Fy_FR"
  Demux1/1 -> Add4/2, Plus1/1  "Fy_FL"
  Demux1/4 -> Add5/2, Plus1/4  "Fy_RR"
  Fy/1 -> Demux1/1
  Plus1/1 -> Add2/2  "sumFy"
  Multiply1/1 -> Add2/1
  Add2/1 -> Ts/M1/1
  Ts/M1/1 -> Add3/2  "delta_Vy"
  Add3/1 -> Mux/2  "Vyk+1"
  Add4/1 -> Multiply2/1
  Constant/1 -> Multiply2/2
  Multiply2/1 -> Add6/1
  Multiply3/1 -> Add6/2
  Constant1/1 -> Multiply3/2
  Add5/1 -> Multiply3/1
  Constant2/1 -> Gain/1
  Gain/1 -> Multiply7/1, Multiply4/2, Multiply5/2, Multiply6/1
  Multiply4/1 -> Add6/3
  Multiply5/1 -> Add6/4
  Multiply6/1 -> Add6/5
  Multiply7/1 -> Add6/6
  Add6/1 -> Ts/Izz/1
  Ts/Izz/1 -> Add7/2  "delta_yawrate"
  Add7/1 -> Mux/3  "yawratek+1"
  statek/1 -> Demux2/1
  Mux/1 -> statek+1/1

== system BAS_MPC_TV/For Iterator Subsystem1/function2/10layer_model/state_k_to_k+8 ==
  Fx : Inport
  Fy : Inport  Port=2
  statek : Inport  Port=3
  Add{,1,3..5,7} (6 alike) : Sum
  Add2 : Sum  Inputs=-+
  Add6 : Sum  Inputs=+--+-+
  Constant : Constant  Value=a
  Constant1 : Constant  Value=b
  Constant2 : Constant  Value=track
  Demux : Demux
  Demux1 : Demux
  Demux2 : Demux  Outputs=3
  Gain : Gain  Gain=0.5
  Multiply{,1..7} (8 alike) : Product
  Mux : Mux  Inputs=3
  Plus : Sum  Inputs=4
  Plus1 : Sum  Inputs=4
  Ts/Izz : Gain  Gain=Ts/Izz
  Ts/M : Gain  Gain=Ts/M
  Ts/M1 : Gain  Gain=Ts/M
  statek+1 : Outport
  wires:
  Demux2/2 -> Add3/1, Multiply/1
  Demux2/3 -> Multiply1/2, Multiply/2, Add7/1
  Multiply/1 -> Add/1
  Add/1 -> Ts/M/1
  Ts/M/1 -> Add1/2  "delta_Vx"
  Demux2/1 -> Add1/1, Multiply1/1
  Add1/1 -> Mux/1  "Vxk+1"
  Fx/1 -> Demux/1
  Demux/1 -> Multiply4/1, Plus/1  "Fx_FL"
  Demux/2 -> Multiply5/1, Plus/2  "Fx_FR"
  Demux/3 -> Multiply6/2, Plus/3  "Fx_RL"
  Demux/4 -> Plus/4, Multiply7/2  "Fx_RR"
  Plus/1 -> Add/2  "sumFx"
  Demux1/3 -> Add5/1, Plus1/3  "Fy_RL"
  Demux1/2 -> Add4/1, Plus1/2  "Fy_FR"
  Demux1/1 -> Add4/2, Plus1/1  "Fy_FL"
  Demux1/4 -> Add5/2, Plus1/4  "Fy_RR"
  Fy/1 -> Demux1/1
  Plus1/1 -> Add2/2  "sumFy"
  Multiply1/1 -> Add2/1
  Add2/1 -> Ts/M1/1
  Ts/M1/1 -> Add3/2  "delta_Vy"
  Add3/1 -> Mux/2  "Vyk+1"
  Add4/1 -> Multiply2/1
  Constant/1 -> Multiply2/2
  Multiply2/1 -> Add6/1
  Multiply3/1 -> Add6/2
  Constant1/1 -> Multiply3/2
  Add5/1 -> Multiply3/1
  Constant2/1 -> Gain/1
  Gain/1 -> Multiply7/1, Multiply4/2, Multiply5/2, Multiply6/1
  Multiply4/1 -> Add6/3
  Multiply5/1 -> Add6/4
  Multiply6/1 -> Add6/5
  Multiply7/1 -> Add6/6
  Add6/1 -> Ts/Izz/1
  Ts/Izz/1 -> Add7/2  "delta_yawrate"
  Add7/1 -> Mux/3  "yawratek+1"
  statek/1 -> Demux2/1
  Mux/1 -> statek+1/1

== system BAS_MPC_TV/For Iterator Subsystem1/function2/10layer_model/state_k_to_k+9 ==
  Fx : Inport
  Fy : Inport  Port=2
  statek : Inport  Port=3
  Add{,1,3..5,7} (6 alike) : Sum
  Add2 : Sum  Inputs=-+
  Add6 : Sum  Inputs=+--+-+
  Constant : Constant  Value=a
  Constant1 : Constant  Value=b
  Constant2 : Constant  Value=track
  Demux : Demux
  Demux1 : Demux
  Demux2 : Demux  Outputs=3
  Gain : Gain  Gain=0.5
  Multiply{,1..7} (8 alike) : Product
  Mux : Mux  Inputs=3
  Plus : Sum  Inputs=4
  Plus1 : Sum  Inputs=4
  Ts/Izz : Gain  Gain=Ts/Izz
  Ts/M : Gain  Gain=Ts/M
  Ts/M1 : Gain  Gain=Ts/M
  statek+1 : Outport
  wires:
  Demux2/2 -> Add3/1, Multiply/1
  Demux2/3 -> Multiply1/2, Multiply/2, Add7/1
  Multiply/1 -> Add/1
  Add/1 -> Ts/M/1
  Ts/M/1 -> Add1/2  "delta_Vx"
  Demux2/1 -> Add1/1, Multiply1/1
  Add1/1 -> Mux/1  "Vxk+1"
  Fx/1 -> Demux/1
  Demux/1 -> Multiply4/1, Plus/1  "Fx_FL"
  Demux/2 -> Multiply5/1, Plus/2  "Fx_FR"
  Demux/3 -> Multiply6/2, Plus/3  "Fx_RL"
  Demux/4 -> Plus/4, Multiply7/2  "Fx_RR"
  Plus/1 -> Add/2  "sumFx"
  Demux1/3 -> Add5/1, Plus1/3  "Fy_RL"
  Demux1/2 -> Add4/1, Plus1/2  "Fy_FR"
  Demux1/1 -> Add4/2, Plus1/1  "Fy_FL"
  Demux1/4 -> Add5/2, Plus1/4  "Fy_RR"
  Fy/1 -> Demux1/1
  Plus1/1 -> Add2/2  "sumFy"
  Multiply1/1 -> Add2/1
  Add2/1 -> Ts/M1/1
  Ts/M1/1 -> Add3/2  "delta_Vy"
  Add3/1 -> Mux/2  "Vyk+1"
  Add4/1 -> Multiply2/1
  Constant/1 -> Multiply2/2
  Multiply2/1 -> Add6/1
  Multiply3/1 -> Add6/2
  Constant1/1 -> Multiply3/2
  Add5/1 -> Multiply3/1
  Constant2/1 -> Gain/1
  Gain/1 -> Multiply7/1, Multiply4/2, Multiply5/2, Multiply6/1
  Multiply4/1 -> Add6/3
  Multiply5/1 -> Add6/4
  Multiply6/1 -> Add6/5
  Multiply7/1 -> Add6/6
  Add6/1 -> Ts/Izz/1
  Ts/Izz/1 -> Add7/2  "delta_yawrate"
  Add7/1 -> Mux/3  "yawratek+1"
  statek/1 -> Demux2/1
  Mux/1 -> statek+1/1

== matlab function BAS_MPC_TV/For Iterator Subsystem1/function/Limitation/MATLAB Function ==
  data: Tl input; y output; T input
function y = fcn(Tl,T)

if (((T(1)+Tl(1))>0)&&((Tl(1)-T(1))>0))
    j1 = 0;
else j1 = 1;
end

if (((T(2)+Tl(2))>0)&&((Tl(2)-T(2))>0))
    j2 = 0;
else j2 = 1;  
end

if (((T(3)+Tl(3))>0)&&((Tl(3)-T(3))>0))
    j3 = 0;
else j3 = 1;
end

if (((T(4)+Tl(4))>0)&&((Tl(4)-T(4))>0))
    j4 = 0;
else j4 = 1;  
end

y = j1+j2+j3+j4;

== matlab function BAS_MPC_TV/For Iterator Subsystem1/MATLAB Function ==
  data: x input; xleft output size=1; dir output size=1; xright output size=1; X output size=1; d input
function [xleft,dir,xright,X] = fcn(x,d)
    
    dir=rands(4,1);
    dir=dir/(eps+norm(dir));
    xleft=x+dir*d;
    xright=x-dir*d;
    X = x;

== matlab function BAS_MPC_TV/convert/MATLAB Function ==
  data: ax input; Fzfl output; ay input; Fzfr output; Fzrl output; Fzrr output
function [Fzfl,Fzfr,Fzrl,Fzrr]  = verticalForce( ax, ay )

% calculate the vertical tire force 
% positive direction
%
%            ↑ ax
%         ←    
%          ay
% 
% 

Mt = 300;
ratio = 0.5;%weight ratio  FRONT/TOTAL
track = 1.2;
wheelbase = 1.5;
Fnf = Mt*0.5*ratio*9.8;
Fnr = Mt*0.5*(1-ratio)*9.8;

Fzfl = Fnf-ax*Mt/wheelbase-ay*Mt/track;
Fzfr = Fnf-ax*Mt/wheelbase+ay*Mt/track;
Fzrl = Fnr+ax*Mt/wheelbase-ay*Mt/track;
Fzrr = Fnr-ax*Mt/wheelbase+ay*Mt/track;

== matlab function BAS_MPC_TV/For Iterator Subsystem1/MATLAB Function1 ==
  data: u1 input; y output; x output; u2 input; u3 input; u4 input
function [y,x]= fcn(u1,u2,u3,u4)

if u1>u2
y = u2;
x = u3;
else
    y = u1;
    x = u4;
end

== matlab function BAS_MPC_TV/convert/MATLAB Function1 ==
  data: Vx0 input; usfl output; Vy0 input; yawrate0 input; usfr output; usrl output; usrr output
function [usfl,usfr,usrl,usrr] = fcn(Vx0,Vy0,yawrate0)

a =1;
b = 0.5;
T = 1.2;
ap = 5;%peak lateral force slip angle
up = 2;%peak lateral coefficient

%%%%无阿克曼 平行转向%%%%%

afl = str-atan((Vy0+a*yawrate0)/(Vx0-T*yawrate0/2));
afr = str-atan((Vy0+a*yawrate0)/(Vx0+T*yawrate0/2));
arl = atan((-Vy0+b*yawrate0)/(Vx0-T*yawrate0/2));
arr = atan((-Vy0+b*yawrate0)/(Vx0+T*yawrate0/02));

usfl = 2*ap*up*afl/(ap^2+afl^2);

usfr = 2*ap*up*afr/(ap^2+afr^2);

usrl = 2*ap*up*arl/(ap^2+arl^2);

usrr = 2*ap*up*arr/(ap^2+arr^2);
